simulink model "Quadrotor_Control"  (R2018b)
settings: Solver=VariableStepAuto  StartTime=0.0  StopTime=32  RelTol=1e-3
values from neighbouring files (symbols this model uses):
  d = 0.086    [lqrparameters.m]    (also in parameters.m = 0.25)
  g = 9.81    [lqrparameters.m]    (also in parameters.m)
  Ix = 0.00025    [lqrparameters.m]    (also in parameters.m)
  Iy = 0.000432    [lqrparameters.m]    (also in parameters.m)
  Iz = 0.0003738    [lqrparameters.m]    (also in parameters.m)
  kftx = 0.1    [lqrparameters.m]
  kfty = 0.1    [lqrparameters.m]
  kftz = 0.1    [lqrparameters.m]
  m = 0.18    [lqrparameters.m]    (also in parameters.m)
undefined symbols (not defined in the file or in its folder): DiscIntNeverNeededParam, K, kfax, kfay, kfaz
libraries: simulink x6
settings Model: Creator=Ayush  LastModifiedBy=Ayush

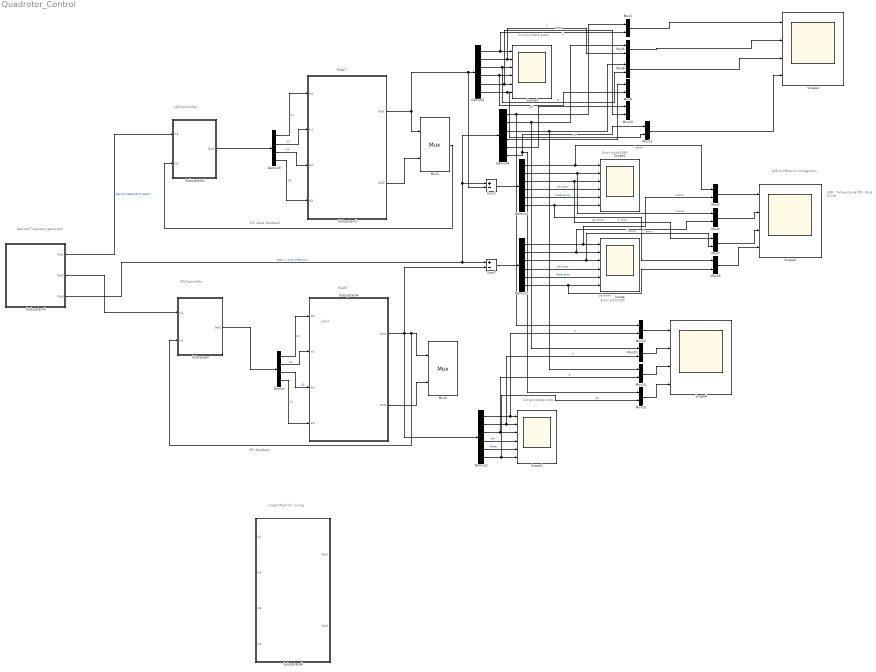
== system Quadrotor_Control ==
  note: Linear Plant for tuning
  note: LQR : Yellow Curve
      | PID : Blue Curve
  note: Desired Trajectory
      | generator
  note: PID
      | Controller
  note: PLANT
  note: Current State
      | plots
  note: PID feedback
  note: Error plots(LQR)
  note: LQR
      | Controller
  note: Full state feedback
  note: PLANT
  note: Current State
      | plots
  note: Error plots(PID)
  note: plant
  note: LQR vs PID
      | error comparison
  Demux : Demux
  Demux{1..2,4..6} (5 alike) : Demux  Outputs=6
  Demux3 : Demux
  Mux{1..16} (16 alike) : Mux  Inputs=2
      Mux1 settings: DisplayOption=signals
      Mux3 settings: DisplayOption=signals
  Scope{,1..3} (4 alike) : Scope  NumInputPorts=6
  Scope4 : Scope  NumInputPorts=4
  Scope5 : Scope  NumInputPorts=4
  Scope6 : Scope  NumInputPorts=4
  Subsystem : Subsystem
  Subsystem1 : Subsystem
  Subsystem2 : Subsystem
  Subsystem3 : Subsystem
  Subsystem4 : Subsystem
  Subsystem6 : Subsystem
  Sum1 : Sum  Inputs=+-
  Sum7 : Sum  Inputs=+-
  wires:
  Mux2/1 -> Scope5/1
  Mux7/1 -> Scope5/3
  Demux5/2 -> Mux6/2, Scope3/2  "Y"
  Demux3/2 -> Subsystem1/2(In1)  "U2"
  Demux5/4 -> Mux9/2, Scope3/4  "phi"
  Subsystem1/1(Out1) -> Mux1/1, Sum1/2, Demux5/1
  Demux4/6 -> Mux16/1, Scope2/6  "psi errror"
  Demux4/1 -> Mux2/1, Scope2/1  "X error"
  Sum1/1 -> Demux4/1
  Mux1/1 -> Subsystem2/2(In2)
  Subsystem2/1(Out1) -> Demux3/1
  Subsystem3/3(Out3) -> Demux6/1, Sum1/1, Sum7/1  "des(x,y,z,phi,theta,psi)"
  Demux3/1 -> Subsystem1/1(In5)  "U1"
  Demux5/3 -> Mux8/2, Scope3/3  "Z"
  Demux1/6 -> Mux16/2, Scope/6  "psi errror"
  Demux1/5 -> Scope/5  "theta error"
  Demux1/2 -> Mux4/2, Scope/2  "Y error"
  Demux3/3 -> Subsystem1/3(In2)  "U3"
  Demux4/5 -> Scope2/5  "theta error"
  Sum7/1 -> Demux1/1
  Mux4/1 -> Scope5/2
  Demux5/1 -> Mux5/2, Scope3/1  "X"
  Demux3/4 -> Subsystem1/4(In3)  "U4"
  Subsystem/1(Out1) -> Demux/1
  Subsystem3/1(Out1) -> Subsystem2/1(In1)  "des full state(12*1 vector)"
  Subsystem4/1(Out1) -> Sum7/2, Demux2/1, Subsystem/2(In2), Mux3/1
  Demux1/1 -> Mux2/2, Scope/1  "X error"
  Demux2/4 -> Scope1/4  "phi"
  Demux4/4 -> Scope2/4  "phi error"
  Demux2/1 -> Mux12/2, Scope1/1  "X"
  Demux4/3 -> Mux7/1, Scope2/3  "Z  error"
  Demux2/5 -> Scope1/5  "theta"
  Demux2/6 -> Mux15/2, Scope1/6  "psi"
  Demux5/6 -> Mux11/2, Scope3/6  "psi"
  Demux2/3 -> Mux14/2, Scope1/3  "Z"
  Demux1/3 -> Mux7/2, Scope/3  "Z  error"
  Demux4/2 -> Mux4/1, Scope2/2  "Y error"
  Demux2/2 -> Mux13/2, Scope1/2  "Y"
  Subsystem4/2(Out2) -> Mux3/2
  Demux1/4 -> Scope/4  "phi error"
  Demux5/5 -> Mux10/2, Scope3/5  "theta"
  Subsystem1/2(Out2) -> Mux1/2
  Demux6/1 -> Mux12/1, Mux5/1
  Demux6/2 -> Mux13/1, Mux6/1
  Demux6/3 -> Mux14/1, Mux8/1
  Demux6/4 -> Mux9/1
  Demux6/5 -> Mux10/1
  Demux6/6 -> Mux15/1, Mux11/1
  Mux6/1 -> Scope4/2
  Mux8/1 -> Scope4/3
  Mux5/1 -> Scope4/1
  Mux11/1 -> Scope4/4
  Mux12/1 -> Scope6/1
  Mux13/1 -> Scope6/2
  Mux14/1 -> Scope6/3
  Mux15/1 -> Scope6/4
  Mux16/1 -> Scope5/4
  Subsystem3/2(Out2) -> Subsystem/1(In1)
  Demux/1 -> Subsystem4/1(In5)  "U1"
  Demux/2 -> Subsystem4/2(In1)  "U2"
  Demux/3 -> Subsystem4/3(In2)  "U3"
  Demux/4 -> Subsystem4/4(In3)  "U4"

== system Quadrotor_Control/Subsystem ==
  note: attitude controller
  note: position controller
  In1 : Inport
  In2 : Inport  Port=2
  Demux : Demux  Outputs=6
  Demux1 : Demux
  Mux2 : Mux
  Subsystem2 : Subsystem
  Subsystem4 : Subsystem  Tag=Position Controller
  Out1 : Outport
  wires:
  Demux/1 -> Subsystem4/5(In5)  "X"
  Subsystem4/3(Out2) -> Subsystem2/1(In1)  "phi commanded"
  Demux1/4 -> Subsystem4/4(In4)  "psi des"
  Demux/5 -> Subsystem2/4(In4)  "theta"
  Subsystem4/4(Out4) -> Mux2/4  "U4"
  Demux1/1 -> Subsystem4/1(In1)  "x des"
  Subsystem4/1(Out3) -> Mux2/1  "U1"
  Subsystem2/1(Out1) -> Mux2/2  "U2"
  Subsystem4/2(Out1) -> Subsystem2/2(In2)  "theta commanded"
  Demux1/2 -> Subsystem4/2(In2)  "y des"
  Mux2/1 -> Out1/1
  Demux/2 -> Subsystem4/6(In6)  "Y"
  Subsystem2/2(Out2) -> Mux2/3  "U3"
  Demux/3 -> Subsystem4/7(In7)  "Z"
  Demux1/3 -> Subsystem4/3(In3)  "z des"
  Demux/4 -> Subsystem2/3(In3)  "phi"
  Demux/6 -> Subsystem4/8(In8)  "psi"
  In2/1 -> Demux/1  "Current State"
  In1/1 -> Demux1/1  "desired(x,y,z,psi)"

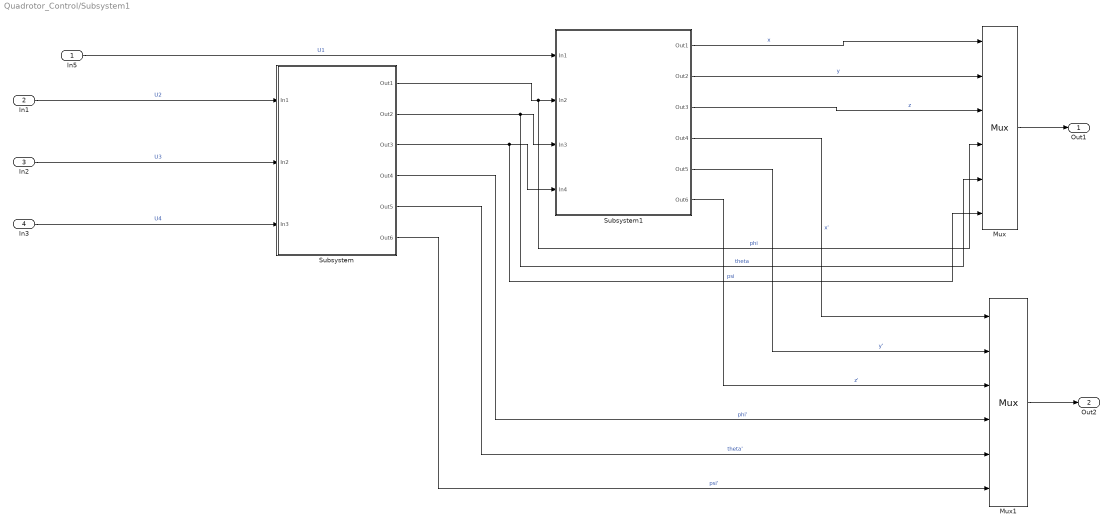
== system Quadrotor_Control/Subsystem1 ==
  In5 : Inport
  In1 : Inport  Port=2
  In2 : Inport  Port=3
  In3 : Inport  Port=4
  Mux : Mux  Inputs=6
      settings: DisplayOption=signals
  Mux1 : Mux  Inputs=6
      settings: DisplayOption=signals
  Subsystem : Subsystem
  Subsystem1 : Subsystem
  Out1 : Outport
  Out2 : Outport  Port=2
  wires:
  Subsystem1/2(Out2) -> Mux/2  "y"
  Subsystem/1(Out1) -> Subsystem1/2(In2), Mux/4  "phi"
  Subsystem1/1(Out1) -> Mux/1  "x"
  In1/1 -> Subsystem/1(In1)  "U2"
  Subsystem/3(Out3) -> Mux/6, Subsystem1/4(In4)  "psi"
  In3/1 -> Subsystem/3(In3)  "U4"
  Subsystem1/3(Out3) -> Mux/3  "z"
  Subsystem1/6(Out6) -> Mux1/3  "z'"
  In2/1 -> Subsystem/2(In2)  "U3"
  In5/1 -> Subsystem1/1(In1)  "U1"
  Subsystem1/4(Out4) -> Mux1/1  "x'"
  Subsystem1/5(Out5) -> Mux1/2  "y'"
  Subsystem/2(Out2) -> Mux/5, Subsystem1/3(In3)  "theta"
  Subsystem/4(Out4) -> Mux1/4  "phi'"
  Subsystem/5(Out5) -> Mux1/5  "theta'"
  Subsystem/6(Out6) -> Mux1/6  "psi'"
  Mux/1 -> Out1/1
  Mux1/1 -> Out2/1

== system Quadrotor_Control/Subsystem2 ==
  In1 : Inport
  In2 : Inport  Port=2
  Gain : Gain  Gain=K  Multiplication=Matrix(K*u)
  Sum : Sum  Inputs=+-
  Out1 : Outport
  wires:
  Sum/1 -> Gain/1
  Gain/1 -> Out1/1
  In1/1 -> Sum/1
  In2/1 -> Sum/2

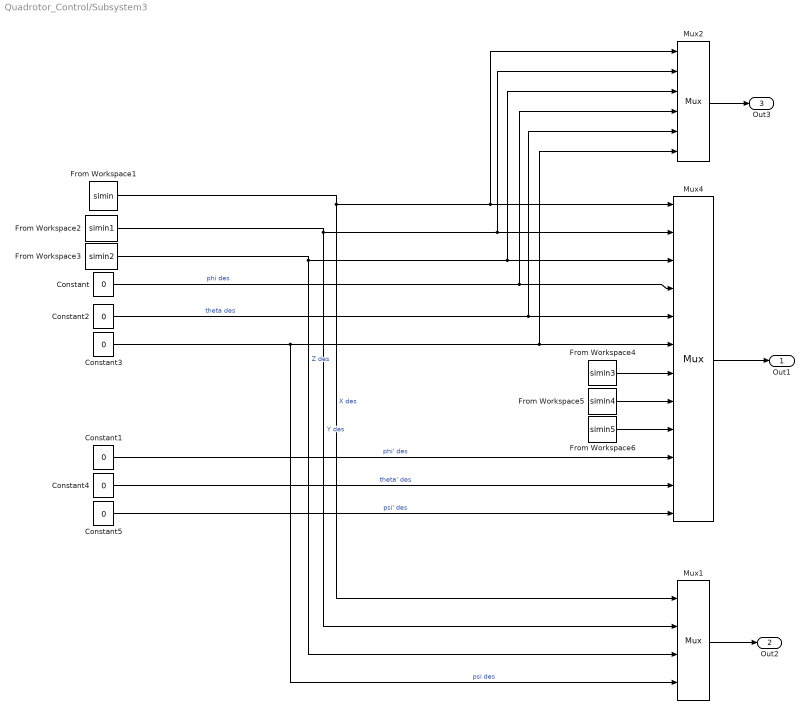
== system Quadrotor_Control/Subsystem3 ==
  Constant{,1..5} (6 alike) : Constant  Value=0
  From Workspace1 : FromWorkspace  VariableName=simin  SampleTime=0.001
  From Workspace2 : FromWorkspace  VariableName=simin1  SampleTime=0.001
  From Workspace3 : FromWorkspace  VariableName=simin2  SampleTime=0.001
  From Workspace4 : FromWorkspace  VariableName=simin3  SampleTime=0.001
  From Workspace5 : FromWorkspace  VariableName=simin4  SampleTime=0.001
  From Workspace6 : FromWorkspace  VariableName=simin5  SampleTime=0.001
  Mux1 : Mux
      settings: DisplayOption=signals
  Mux2 : Mux  Inputs=6
      settings: DisplayOption=signals
  Mux4 : Mux  Inputs=12
      settings: DisplayOption=signals
  Out1 : Outport
  Out2 : Outport  Port=2
  Out3 : Outport  Port=3
  wires:
  From Workspace1/1 -> Mux1/1, Mux2/1, Mux4/1  "X des"
  Constant1/1 -> Mux4/10  "phi' des"
  From Workspace2/1 -> Mux1/2, Mux2/2, Mux4/2  "Y des"
  Constant2/1 -> Mux2/5, Mux4/5  "theta des"
  Constant/1 -> Mux2/4, Mux4/4  "phi des"
  Constant5/1 -> Mux4/12  "psi' des"
  From Workspace3/1 -> Mux1/3, Mux2/3, Mux4/3  "Z des"
  Constant3/1 -> Mux1/4, Mux2/6, Mux4/6  "psi des"
  Constant4/1 -> Mux4/11  "theta' des"
  Mux1/1 -> Out2/1
  Mux4/1 -> Out1/1
  Mux2/1 -> Out3/1
  From Workspace4/1 -> Mux4/7
  From Workspace5/1 -> Mux4/8
  From Workspace6/1 -> Mux4/9

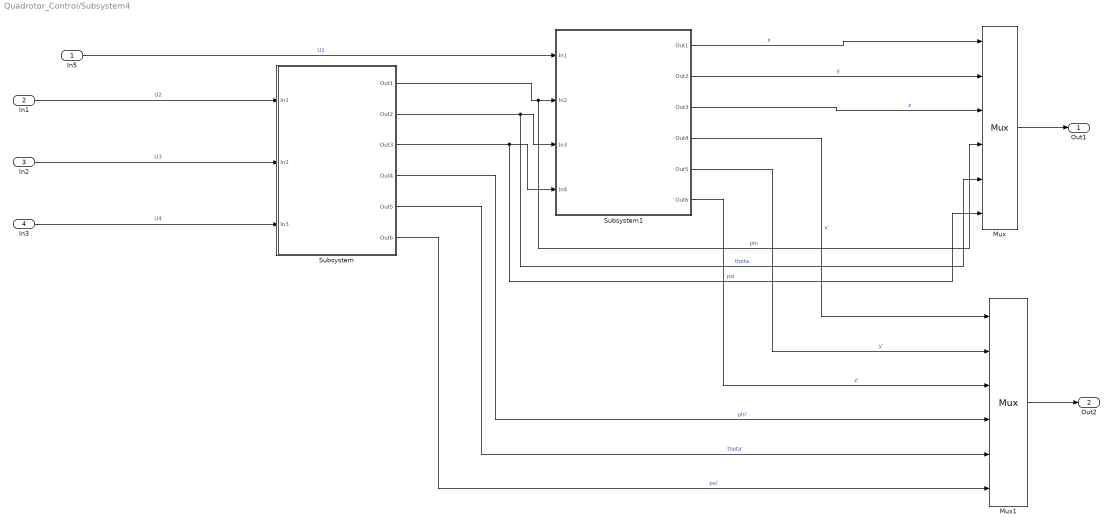
== system Quadrotor_Control/Subsystem4 ==
  In5 : Inport
  In1 : Inport  Port=2
  In2 : Inport  Port=3
  In3 : Inport  Port=4
  Mux : Mux  Inputs=6
      settings: DisplayOption=signals
  Mux1 : Mux  Inputs=6
      settings: DisplayOption=signals
  Subsystem : Subsystem
  Subsystem1 : Subsystem
  Out1 : Outport
  Out2 : Outport  Port=2
  wires:
  Subsystem1/2(Out2) -> Mux/2  "y"
  Subsystem/1(Out1) -> Subsystem1/2(In2), Mux/4  "phi"
  Subsystem1/1(Out1) -> Mux/1  "x"
  In1/1 -> Subsystem/1(In1)  "U2"
  Subsystem/3(Out3) -> Mux/6, Subsystem1/4(In4)  "psi"
  In3/1 -> Subsystem/3(In3)  "U4"
  Subsystem1/3(Out3) -> Mux/3  "z"
  Subsystem1/6(Out6) -> Mux1/3  "z'"
  In2/1 -> Subsystem/2(In2)  "U3"
  In5/1 -> Subsystem1/1(In1)  "U1"
  Subsystem1/4(Out4) -> Mux1/1  "x'"
  Subsystem1/5(Out5) -> Mux1/2  "y'"
  Subsystem/2(Out2) -> Mux/5, Subsystem1/3(In3)  "theta"
  Subsystem/4(Out4) -> Mux1/4  "phi'"
  Subsystem/5(Out5) -> Mux1/5  "theta'"
  Subsystem/6(Out6) -> Mux1/6  "psi'"
  Mux/1 -> Out1/1
  Mux1/1 -> Out2/1

== system Quadrotor_Control/Subsystem6 ==
  note: State Vector
      | Derivative
  note: State Vector
  In1 : Inport
  In2 : Inport  Port=2
  In3 : Inport  Port=3
  In4 : Inport  Port=4
  Mux1 : Mux  Inputs=6
      settings: DisplayOption=signals
  Mux3 : Mux  Inputs=6
      settings: DisplayOption=signals
  Subsystem1 : Subsystem
  Subsystem2 : Subsystem
  Out1 : Outport
  Out2 : Outport  Port=2
  wires:
  Subsystem1/1(Out1) -> Mux3/4, Subsystem2/2(In2)  "phi"
  Subsystem2/6(Out6) -> Mux1/3  "Z'"
  Subsystem2/5(Out5) -> Mux1/2  "Y'"
  Subsystem2/1(Out1) -> Mux3/1  "X"
  Subsystem1/2(Out2) -> Mux3/5, Subsystem2/3(In3)  "theta"
  Subsystem1/3(Out3) -> Mux3/6  "psi"
  Subsystem2/4(Out4) -> Mux1/1  "X'"
  Subsystem2/3(Out3) -> Mux3/3  "Z"
  In4/1 -> Subsystem1/3(In3)  "U4"
  In3/1 -> Subsystem1/2(In2)  "U3"
  Subsystem2/2(Out2) -> Mux3/2  "Y"
  In2/1 -> Subsystem1/1(In1)  "U2"
  In1/1 -> Subsystem2/1(In1)  "U1"
  Subsystem1/4(Out4) -> Mux1/4  "phi'"
  Subsystem1/5(Out5) -> Mux1/5  "theta'"
  Subsystem1/6(Out6) -> Mux1/6  "psi'"
  Mux1/1 -> Out2/1  "X' (State Derivative)"
  Mux3/1 -> Out1/1  "X(state Vector)"

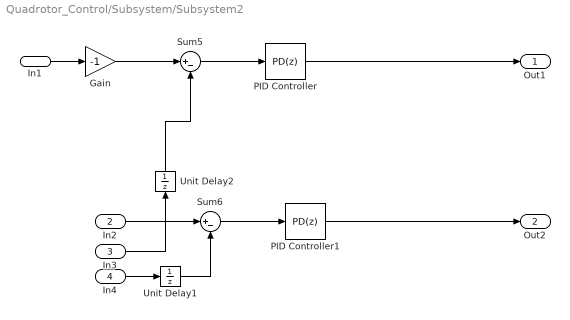
== system Quadrotor_Control/Subsystem/Subsystem2 ==
  In1 : Inport
  In2 : Inport  Port=2
  In3 : Inport  Port=3
  In4 : Inport  Port=4
  Gain : Gain  Gain=-1
  PID Controller : simulink/Continuous/PID Controller  Controller=PD  Form=Parallel  TimeDomain=Discrete-time  SampleTime=0.001  IntegratorMethod=Forward Euler  FilterMethod=Forward Euler  ControllerParametersSource=internal  P=0.492  I=0.1  D=0.08414  UseFilter=off  N=100  TunerSelectOption=Transfer Function Based (PID Tuner App)  InitialConditionSource=internal  InitialConditionForIntegrator=0  InitialConditionForFilter=0  DifferentiatorICPrevScaledInput=0  ExternalReset=none  TrackingMode=off  Kt=1  LimitOutput=off  UpperSaturationLimit=inf  LowerSaturationLimit=-inf  LinearizeAsGain=on  AntiWindupMode=none  Kb=1  POutMin=[]  POutMax=[]  IOutMin=[]  IOutMax=[]  DOutMin=[]  DOutMax=[]  NOutMin=[]  NOutMax=[]  SumOutMin=[]  SumOutMax=[]  SaturationOutMin=[]  SaturationOutMax=[]  PParamMin=[]  PParamMax=[]  IParamMin=[]  IParamMax=[]  DParamMin=[]  DParamMax=[]  NParamMin=[]  NParamMax=[]  KbParamMin=[]  KbParamMax=[]  KtParamMin=[]  KtParamMax=[]  KbOutMin=[]  KbOutMax=[]  KtOutMin=[]  KtOutMax=[]  IntegratorOutMin=[]  IntegratorOutMax=[]  FilterOutMin=[]  FilterOutMax=[]  SumI1OutMin=[]  SumI1OutMax=[]  SumI2OutMin=[]  SumI2OutMax=[]  SumI3OutMin=[]  SumI3OutMax=[]  SumI4OutMin=[]  SumI4OutMax=[]  SumDOutMin=[]  SumDOutMax=[]  DifferentiatorOutMin=[]  DifferentiatorOutMax=[]  FilterDiffOutCoefMin=[]  FilterDiffOutCoefMax=[]  ReciprocalOutMin=[]  ReciprocalOutMax=[]  SumDenOutMin=[]  SumDenOutMax=[]  SumNumOutMin=[]  SumNumOutMax=[]  DivideOutMin=[]  DivideOutMax=[]  IntegratorContinuousStateAttributes=''  IntegratorStateMustResolveToSignalObject=off  IntegratorRTWStateStorageClass=Auto  FilterContinuousStateAttributes=''  FilterStateMustResolveToSignalObject=off  FilterRTWStateStorageClass=Auto  ParallelPVariant=InternalParameters  IdealPVariant=Disabled  IVariant=Disabled  DVariant=InternalParameters  IntegratorVariant=Disabled  SatVariant=Disabled  AWVariant=Disabled  PCopyVariant=Disabled  TRVariant=Disabled  FdbkBlocksVariant=Forward  IdealPFdbkVariant=Disabled  SatFdbkVariant=Disabled  DerivativeFilterVariant=Differentiator  NVariant=Passthrough  NCopyVariant=Disabled_SignalSpec  FilterICVariant=InternalICsDifferentiator  IntegratorICVariant=Disabled  ExternalResetVariant=Disabled  TRSumVariant=Passthrough  SumFdbkVariant=Disabled  SumVariant=Sum_PD
  PID Controller1 : simulink/Continuous/PID Controller  Controller=PD  Form=Parallel  TimeDomain=Discrete-time  SampleTime=0.001  IntegratorMethod=Forward Euler  FilterMethod=Forward Euler  ControllerParametersSource=internal  P=0.7754  I=1  D=0.1389  UseFilter=off  N=100  TunerSelectOption=Transfer Function Based (PID Tuner App)  InitialConditionSource=internal  InitialConditionForIntegrator=0  InitialConditionForFilter=0  DifferentiatorICPrevScaledInput=0  ExternalReset=none  TrackingMode=off  Kt=1  LimitOutput=off  UpperSaturationLimit=inf  LowerSaturationLimit=-inf  LinearizeAsGain=on  AntiWindupMode=none  Kb=1  POutMin=[]  POutMax=[]  IOutMin=[]  IOutMax=[]  DOutMin=[]  DOutMax=[]  NOutMin=[]  NOutMax=[]  SumOutMin=[]  SumOutMax=[]  SaturationOutMin=[]  SaturationOutMax=[]  PParamMin=[]  PParamMax=[]  IParamMin=[]  IParamMax=[]  DParamMin=[]  DParamMax=[]  NParamMin=[]  NParamMax=[]  KbParamMin=[]  KbParamMax=[]  KtParamMin=[]  KtParamMax=[]  KbOutMin=[]  KbOutMax=[]  KtOutMin=[]  KtOutMax=[]  IntegratorOutMin=[]  IntegratorOutMax=[]  FilterOutMin=[]  FilterOutMax=[]  SumI1OutMin=[]  SumI1OutMax=[]  SumI2OutMin=[]  SumI2OutMax=[]  SumI3OutMin=[]  SumI3OutMax=[]  SumI4OutMin=[]  SumI4OutMax=[]  SumDOutMin=[]  SumDOutMax=[]  DifferentiatorOutMin=[]  DifferentiatorOutMax=[]  FilterDiffOutCoefMin=[]  FilterDiffOutCoefMax=[]  ReciprocalOutMin=[]  ReciprocalOutMax=[]  SumDenOutMin=[]  SumDenOutMax=[]  SumNumOutMin=[]  SumNumOutMax=[]  DivideOutMin=[]  DivideOutMax=[]  IntegratorContinuousStateAttributes=''  IntegratorStateMustResolveToSignalObject=off  IntegratorRTWStateStorageClass=Auto  FilterContinuousStateAttributes=''  FilterStateMustResolveToSignalObject=off  FilterRTWStateStorageClass=Auto  ParallelPVariant=InternalParameters  IdealPVariant=Disabled  IVariant=Disabled  DVariant=InternalParameters  IntegratorVariant=Disabled  SatVariant=Disabled  AWVariant=Disabled  PCopyVariant=Disabled  TRVariant=Disabled  FdbkBlocksVariant=Forward  IdealPFdbkVariant=Disabled  SatFdbkVariant=Disabled  DerivativeFilterVariant=Differentiator  NVariant=Passthrough  NCopyVariant=Disabled_SignalSpec  FilterICVariant=InternalICsDifferentiator  IntegratorICVariant=Disabled  ExternalResetVariant=Disabled  TRSumVariant=Passthrough  SumFdbkVariant=Disabled  SumVariant=Sum_PD
  Sum5 : Sum  Inputs=|+-
  Sum6 : Sum  Inputs=|+-
  Unit Delay1 : UnitDelay  SampleTime=0.001
  Unit Delay2 : UnitDelay  SampleTime=0.001
  Out1 : Outport
  Out2 : Outport  Port=2
  wires:
  Sum6/1 -> PID Controller1/1
  PID Controller1/1 -> Out2/1
  In2/1 -> Sum6/1
  In4/1 -> Unit Delay1/1
  Unit Delay1/1 -> Sum6/2
  PID Controller/1 -> Out1/1
  Sum5/1 -> PID Controller/1
  In1/1 -> Gain/1
  Gain/1 -> Sum5/1
  In3/1 -> Unit Delay2/1
  Unit Delay2/1 -> Sum5/2

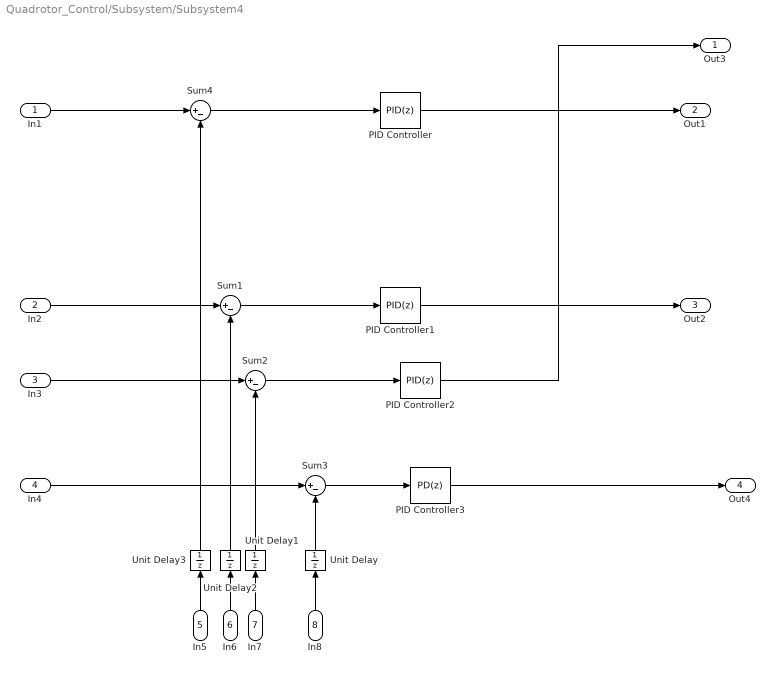
== system Quadrotor_Control/Subsystem/Subsystem4 ==
  In1 : Inport
  In2 : Inport  Port=2
  In3 : Inport  Port=3
  In4 : Inport  Port=4
  In5 : Inport  Port=5
  In6 : Inport  Port=6
  In7 : Inport  Port=7
  In8 : Inport  Port=8
  PID Controller : simulink/Continuous/PID Controller  Controller=PID  Form=Parallel  TimeDomain=Discrete-time  SampleTime=0.001  IntegratorMethod=Forward Euler  FilterMethod=Forward Euler  ControllerParametersSource=internal  P=0.4475  I=0.0442  D=1.133  UseFilter=off  N=100  TunerSelectOption=Transfer Function Based (PID Tuner App)  InitialConditionSource=internal  InitialConditionForIntegrator=0  InitialConditionForFilter=0  DifferentiatorICPrevScaledInput=0  ExternalReset=none  TrackingMode=off  Kt=1  LimitOutput=off  UpperSaturationLimit=inf  LowerSaturationLimit=-inf  LinearizeAsGain=on  AntiWindupMode=none  Kb=1  POutMin=[]  POutMax=[]  IOutMin=[]  IOutMax=[]  DOutMin=[]  DOutMax=[]  NOutMin=[]  NOutMax=[]  SumOutMin=[]  SumOutMax=[]  SaturationOutMin=[]  SaturationOutMax=[]  PParamMin=[]  PParamMax=[]  IParamMin=[]  IParamMax=[]  DParamMin=[]  DParamMax=[]  NParamMin=[]  NParamMax=[]  KbParamMin=[]  KbParamMax=[]  KtParamMin=[]  KtParamMax=[]  KbOutMin=[]  KbOutMax=[]  KtOutMin=[]  KtOutMax=[]  IntegratorOutMin=[]  IntegratorOutMax=[]  FilterOutMin=[]  FilterOutMax=[]  SumI1OutMin=[]  SumI1OutMax=[]  SumI2OutMin=[]  SumI2OutMax=[]  SumI3OutMin=[]  SumI3OutMax=[]  SumI4OutMin=[]  SumI4OutMax=[]  SumDOutMin=[]  SumDOutMax=[]  DifferentiatorOutMin=[]  DifferentiatorOutMax=[]  FilterDiffOutCoefMin=[]  FilterDiffOutCoefMax=[]  ReciprocalOutMin=[]  ReciprocalOutMax=[]  SumDenOutMin=[]  SumDenOutMax=[]  SumNumOutMin=[]  SumNumOutMax=[]  DivideOutMin=[]  DivideOutMax=[]  IntegratorContinuousStateAttributes=''  IntegratorStateMustResolveToSignalObject=off  IntegratorRTWStateStorageClass=Auto  FilterContinuousStateAttributes=''  FilterStateMustResolveToSignalObject=off  FilterRTWStateStorageClass=Auto  ParallelPVariant=InternalParameters  IdealPVariant=Disabled  IVariant=InternalParameters  DVariant=InternalParameters  IntegratorVariant=Discrete  SatVariant=Disabled  AWVariant=Passthrough  PCopyVariant=Disabled  TRVariant=Disabled  FdbkBlocksVariant=Forward  IdealPFdbkVariant=Disabled  SatFdbkVariant=Disabled  DerivativeFilterVariant=Differentiator  NVariant=Passthrough  NCopyVariant=Disabled_SignalSpec  FilterICVariant=InternalICsDifferentiator  IntegratorICVariant=InternalICs  ExternalResetVariant=Disabled  TRSumVariant=Passthrough  SumFdbkVariant=Disabled  SumVariant=Sum_PID
  PID Controller1 : simulink/Continuous/PID Controller  Controller=PID  Form=Parallel  TimeDomain=Discrete-time  SampleTime=0.001  IntegratorMethod=Forward Euler  FilterMethod=Forward Euler  ControllerParametersSource=internal  P=0.4473  I=0.04417  D=1.133  UseFilter=off  N=100  TunerSelectOption=Transfer Function Based (PID Tuner App)  InitialConditionSource=internal  InitialConditionForIntegrator=0  InitialConditionForFilter=0  DifferentiatorICPrevScaledInput=0  ExternalReset=none  TrackingMode=off  Kt=1  LimitOutput=off  UpperSaturationLimit=inf  LowerSaturationLimit=-inf  LinearizeAsGain=on  AntiWindupMode=none  Kb=1  POutMin=[]  POutMax=[]  IOutMin=[]  IOutMax=[]  DOutMin=[]  DOutMax=[]  NOutMin=[]  NOutMax=[]  SumOutMin=[]  SumOutMax=[]  SaturationOutMin=[]  SaturationOutMax=[]  PParamMin=[]  PParamMax=[]  IParamMin=[]  IParamMax=[]  DParamMin=[]  DParamMax=[]  NParamMin=[]  NParamMax=[]  KbParamMin=[]  KbParamMax=[]  KtParamMin=[]  KtParamMax=[]  KbOutMin=[]  KbOutMax=[]  KtOutMin=[]  KtOutMax=[]  IntegratorOutMin=[]  IntegratorOutMax=[]  FilterOutMin=[]  FilterOutMax=[]  SumI1OutMin=[]  SumI1OutMax=[]  SumI2OutMin=[]  SumI2OutMax=[]  SumI3OutMin=[]  SumI3OutMax=[]  SumI4OutMin=[]  SumI4OutMax=[]  SumDOutMin=[]  SumDOutMax=[]  DifferentiatorOutMin=[]  DifferentiatorOutMax=[]  FilterDiffOutCoefMin=[]  FilterDiffOutCoefMax=[]  ReciprocalOutMin=[]  ReciprocalOutMax=[]  SumDenOutMin=[]  SumDenOutMax=[]  SumNumOutMin=[]  SumNumOutMax=[]  DivideOutMin=[]  DivideOutMax=[]  IntegratorContinuousStateAttributes=''  IntegratorStateMustResolveToSignalObject=off  IntegratorRTWStateStorageClass=Auto  FilterContinuousStateAttributes=''  FilterStateMustResolveToSignalObject=off  FilterRTWStateStorageClass=Auto  ParallelPVariant=InternalParameters  IdealPVariant=Disabled  IVariant=InternalParameters  DVariant=InternalParameters  IntegratorVariant=Discrete  SatVariant=Disabled  AWVariant=Passthrough  PCopyVariant=Disabled  TRVariant=Disabled  FdbkBlocksVariant=Forward  IdealPFdbkVariant=Disabled  SatFdbkVariant=Disabled  DerivativeFilterVariant=Differentiator  NVariant=Passthrough  NCopyVariant=Disabled_SignalSpec  FilterICVariant=InternalICsDifferentiator  IntegratorICVariant=InternalICs  ExternalResetVariant=Disabled  TRSumVariant=Passthrough  SumFdbkVariant=Disabled  SumVariant=Sum_PID
  PID Controller2 : simulink/Continuous/PID Controller  Controller=PID  Form=Parallel  TimeDomain=Discrete-time  SampleTime=0.001  IntegratorMethod=Forward Euler  FilterMethod=Forward Euler  ControllerParametersSource=internal  P=0.8029  I=0.07931  D=2.032  UseFilter=off  N=100  TunerSelectOption=Transfer Function Based (PID Tuner App)  InitialConditionSource=internal  InitialConditionForIntegrator=0  InitialConditionForFilter=0  DifferentiatorICPrevScaledInput=0  ExternalReset=none  TrackingMode=off  Kt=1  LimitOutput=off  UpperSaturationLimit=inf  LowerSaturationLimit=-inf  LinearizeAsGain=on  AntiWindupMode=none  Kb=1  POutMin=[]  POutMax=[]  IOutMin=[]  IOutMax=[]  DOutMin=[]  DOutMax=[]  NOutMin=[]  NOutMax=[]  SumOutMin=[]  SumOutMax=[]  SaturationOutMin=[]  SaturationOutMax=[]  PParamMin=[]  PParamMax=[]  IParamMin=[]  IParamMax=[]  DParamMin=[]  DParamMax=[]  NParamMin=[]  NParamMax=[]  KbParamMin=[]  KbParamMax=[]  KtParamMin=[]  KtParamMax=[]  KbOutMin=[]  KbOutMax=[]  KtOutMin=[]  KtOutMax=[]  IntegratorOutMin=[]  IntegratorOutMax=[]  FilterOutMin=[]  FilterOutMax=[]  SumI1OutMin=[]  SumI1OutMax=[]  SumI2OutMin=[]  SumI2OutMax=[]  SumI3OutMin=[]  SumI3OutMax=[]  SumI4OutMin=[]  SumI4OutMax=[]  SumDOutMin=[]  SumDOutMax=[]  DifferentiatorOutMin=[]  DifferentiatorOutMax=[]  FilterDiffOutCoefMin=[]  FilterDiffOutCoefMax=[]  ReciprocalOutMin=[]  ReciprocalOutMax=[]  SumDenOutMin=[]  SumDenOutMax=[]  SumNumOutMin=[]  SumNumOutMax=[]  DivideOutMin=[]  DivideOutMax=[]  IntegratorContinuousStateAttributes=''  IntegratorStateMustResolveToSignalObject=off  IntegratorRTWStateStorageClass=Auto  FilterContinuousStateAttributes=''  FilterStateMustResolveToSignalObject=off  FilterRTWStateStorageClass=Auto  ParallelPVariant=InternalParameters  IdealPVariant=Disabled  IVariant=InternalParameters  DVariant=InternalParameters  IntegratorVariant=Discrete  SatVariant=Disabled  AWVariant=Passthrough  PCopyVariant=Disabled  TRVariant=Disabled  FdbkBlocksVariant=Forward  IdealPFdbkVariant=Disabled  SatFdbkVariant=Disabled  DerivativeFilterVariant=Differentiator  NVariant=Passthrough  NCopyVariant=Disabled_SignalSpec  FilterICVariant=InternalICsDifferentiator  IntegratorICVariant=InternalICs  ExternalResetVariant=Disabled  TRSumVariant=Passthrough  SumFdbkVariant=Disabled  SumVariant=Sum_PID
  PID Controller3 : simulink/Continuous/PID Controller  Controller=PD  Form=Parallel  TimeDomain=Discrete-time  SampleTime=0.001  IntegratorMethod=Forward Euler  FilterMethod=Forward Euler  ControllerParametersSource=internal  P=0.546  I=1  D=0.1077  UseFilter=off  N=100  TunerSelectOption=Transfer Function Based (PID Tuner App)  InitialConditionSource=internal  InitialConditionForIntegrator=0  InitialConditionForFilter=0  DifferentiatorICPrevScaledInput=0  ExternalReset=none  TrackingMode=off  Kt=1  LimitOutput=off  UpperSaturationLimit=inf  LowerSaturationLimit=-inf  LinearizeAsGain=on  AntiWindupMode=none  Kb=1  POutMin=[]  POutMax=[]  IOutMin=[]  IOutMax=[]  DOutMin=[]  DOutMax=[]  NOutMin=[]  NOutMax=[]  SumOutMin=[]  SumOutMax=[]  SaturationOutMin=[]  SaturationOutMax=[]  PParamMin=[]  PParamMax=[]  IParamMin=[]  IParamMax=[]  DParamMin=[]  DParamMax=[]  NParamMin=[]  NParamMax=[]  KbParamMin=[]  KbParamMax=[]  KtParamMin=[]  KtParamMax=[]  KbOutMin=[]  KbOutMax=[]  KtOutMin=[]  KtOutMax=[]  IntegratorOutMin=[]  IntegratorOutMax=[]  FilterOutMin=[]  FilterOutMax=[]  SumI1OutMin=[]  SumI1OutMax=[]  SumI2OutMin=[]  SumI2OutMax=[]  SumI3OutMin=[]  SumI3OutMax=[]  SumI4OutMin=[]  SumI4OutMax=[]  SumDOutMin=[]  SumDOutMax=[]  DifferentiatorOutMin=[]  DifferentiatorOutMax=[]  FilterDiffOutCoefMin=[]  FilterDiffOutCoefMax=[]  ReciprocalOutMin=[]  ReciprocalOutMax=[]  SumDenOutMin=[]  SumDenOutMax=[]  SumNumOutMin=[]  SumNumOutMax=[]  DivideOutMin=[]  DivideOutMax=[]  IntegratorContinuousStateAttributes=''  IntegratorStateMustResolveToSignalObject=off  IntegratorRTWStateStorageClass=Auto  FilterContinuousStateAttributes=''  FilterStateMustResolveToSignalObject=off  FilterRTWStateStorageClass=Auto  ParallelPVariant=InternalParameters  IdealPVariant=Disabled  IVariant=Disabled  DVariant=InternalParameters  IntegratorVariant=Disabled  SatVariant=Disabled  AWVariant=Disabled  PCopyVariant=Disabled  TRVariant=Disabled  FdbkBlocksVariant=Forward  IdealPFdbkVariant=Disabled  SatFdbkVariant=Disabled  DerivativeFilterVariant=Differentiator  NVariant=Passthrough  NCopyVariant=Disabled_SignalSpec  FilterICVariant=InternalICsDifferentiator  IntegratorICVariant=Disabled  ExternalResetVariant=Disabled  TRSumVariant=Passthrough  SumFdbkVariant=Disabled  SumVariant=Sum_PD
  Sum{1..4} (4 alike) : Sum  Inputs=|+-
  Unit Delay{,1..3} (4 alike) : UnitDelay  SampleTime=0.001
  Out3 : Outport
  Out1 : Outport  Port=2
  Out2 : Outport  Port=3
  Out4 : Outport  Port=4
  wires:
  PID Controller3/1 -> Out4/1
  In7/1 -> Unit Delay1/1
  In6/1 -> Unit Delay2/1
  In8/1 -> Unit Delay/1
  In5/1 -> Unit Delay3/1
  Unit Delay2/1 -> Sum1/2
  Sum1/1 -> PID Controller1/1
  Unit Delay1/1 -> Sum2/2
  Sum3/1 -> PID Controller3/1
  PID Controller1/1 -> Out2/1
  PID Controller2/1 -> Out3/1
  Sum2/1 -> PID Controller2/1
  Unit Delay/1 -> Sum3/2
  PID Controller/1 -> Out1/1
  Sum4/1 -> PID Controller/1
  Unit Delay3/1 -> Sum4/2
  In1/1 -> Sum4/1
  In2/1 -> Sum1/1
  In3/1 -> Sum2/1
  In4/1 -> Sum3/1

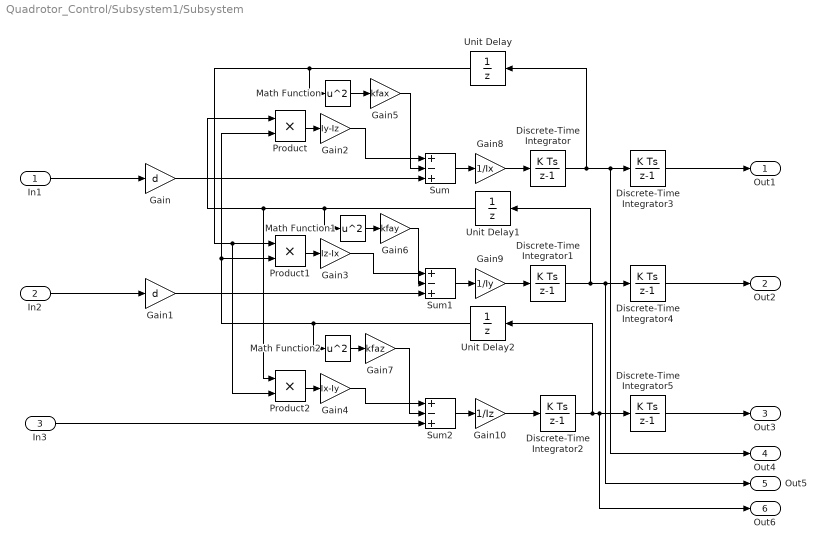
== system Quadrotor_Control/Subsystem1/Subsystem ==
  In1 : Inport
  In2 : Inport  Port=2
  In3 : Inport  Port=3
  Discrete-Time Integrator{,1..5} (6 alike) : DiscreteIntegrator  SampleTime=-1  ICPrevOutput=DiscIntNeverNeededParam  ICPrevScaledInput=DiscIntNeverNeededParam
  Gain : Gain  Gain=d
  Gain1 : Gain  Gain=d
  Gain10 : Gain  Gain=1/Iz
  Gain2 : Gain  Gain=Iy-Iz
  Gain3 : Gain  Gain=Iz-Ix
  Gain4 : Gain  Gain=Ix-Iy
  Gain5 : Gain  Gain=kfax
  Gain6 : Gain  Gain=kfay
  Gain7 : Gain  Gain=kfaz
  Gain8 : Gain  Gain=1/Ix
  Gain9 : Gain  Gain=1/Iy
  Math Function : Math  Operator=square  SaturateOnIntegerOverflow=on
  Math Function1 : Math  Operator=square  SaturateOnIntegerOverflow=on
  Math Function2 : Math  Operator=square  SaturateOnIntegerOverflow=on
  Product : Product
  Product1 : Product
  Product2 : Product
  Sum : Sum  Inputs=+-+
  Sum1 : Sum  Inputs=+-+
  Sum2 : Sum  Inputs=+-+
  Unit Delay : UnitDelay  SampleTime=0.001
  Unit Delay1 : UnitDelay  SampleTime=0.001
  Unit Delay2 : UnitDelay  SampleTime=0.001
  Out1 : Outport
  Out2 : Outport  Port=2
  Out3 : Outport  Port=3
  Out4 : Outport  Port=4
  Out5 : Outport  Port=5
  Out6 : Outport  Port=6
  wires:
  Unit Delay/1 -> Math Function/1, Product2/2, Product1/1
  Discrete-Time Integrator1/1 -> Out5/1, Discrete-Time Integrator4/1, Unit Delay1/1
  Unit Delay1/1 -> Math Function1/1, Product2/1, Product/1
  Discrete-Time Integrator2/1 -> Out6/1, Discrete-Time Integrator5/1, Unit Delay2/1
  Unit Delay2/1 -> Math Function2/1, Product1/2, Product/2
  Product1/1 -> Gain3/1
  Discrete-Time Integrator/1 -> Out4/1, Discrete-Time Integrator3/1, Unit Delay/1
  Gain10/1 -> Discrete-Time Integrator2/1
  Discrete-Time Integrator3/1 -> Out1/1
  Gain4/1 -> Sum2/1
  Gain/1 -> Sum/3
  Discrete-Time Integrator4/1 -> Out2/1
  Math Function/1 -> Gain5/1
  Gain5/1 -> Sum/2
  Product/1 -> Gain2/1
  Math Function1/1 -> Gain6/1
  Gain6/1 -> Sum1/2
  Gain7/1 -> Sum2/2
  Gain2/1 -> Sum/1
  Math Function2/1 -> Gain7/1
  Sum2/1 -> Gain10/1
  Gain9/1 -> Discrete-Time Integrator1/1
  Gain8/1 -> Discrete-Time Integrator/1
  Sum/1 -> Gain8/1
  Gain3/1 -> Sum1/1
  Product2/1 -> Gain4/1
  Gain1/1 -> Sum1/3
  Sum1/1 -> Gain9/1
  Discrete-Time Integrator5/1 -> Out3/1
  In1/1 -> Gain/1
  In2/1 -> Gain1/1
  In3/1 -> Sum2/3

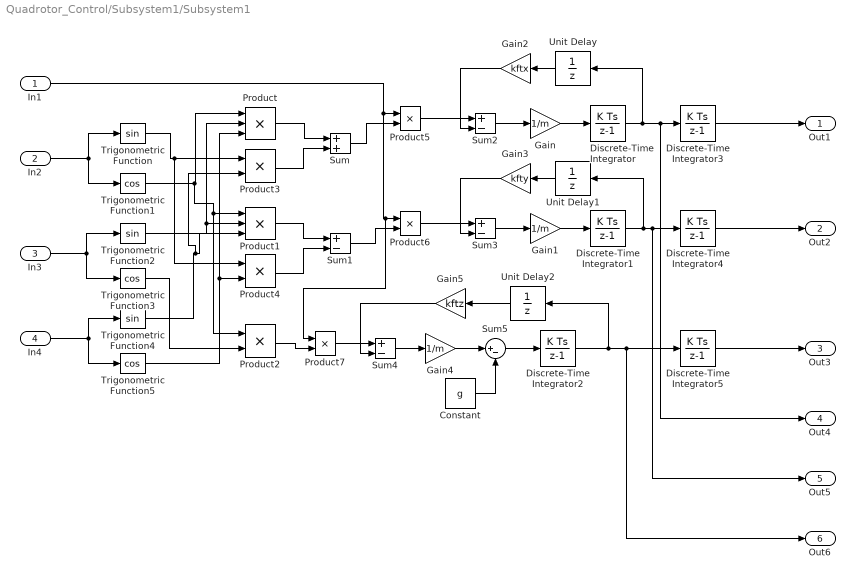
== system Quadrotor_Control/Subsystem1/Subsystem1 ==
  In1 : Inport
  In2 : Inport  Port=2
  In3 : Inport  Port=3
  In4 : Inport  Port=4
  Constant : Constant  Value=g
  Discrete-Time Integrator{,1..5} (6 alike) : DiscreteIntegrator  SampleTime=0.001  ICPrevOutput=DiscIntNeverNeededParam  ICPrevScaledInput=DiscIntNeverNeededParam
  Gain : Gain  Gain=1/m
  Gain1 : Gain  Gain=1/m
  Gain2 : Gain  Gain=kftx
  Gain3 : Gain  Gain=kfty
  Gain4 : Gain  Gain=1/m
  Gain5 : Gain  Gain=kftz
  Product : Product  Inputs=3
  Product1 : Product  Inputs=3
  Product{2..7} (6 alike) : Product
  Sum : Sum
  Sum{1..4} (4 alike) : Sum  Inputs=+-
  Sum5 : Sum  Inputs=|+-
  Trigonometric Function : Trigonometry
  Trigonometric Function1 : Trigonometry  Operator=cos
  Trigonometric Function2 : Trigonometry
  Trigonometric Function3 : Trigonometry  Operator=cos
  Trigonometric Function4 : Trigonometry
  Trigonometric Function5 : Trigonometry  Operator=cos
  Unit Delay : UnitDelay  SampleTime=0.001
  Unit Delay1 : UnitDelay  SampleTime=0.001
  Unit Delay2 : UnitDelay  SampleTime=0.001
  Out1 : Outport
  Out2 : Outport  Port=2
  Out3 : Outport  Port=3
  Out4 : Outport  Port=4
  Out5 : Outport  Port=5
  Out6 : Outport  Port=6
  wires:
  Sum2/1 -> Gain/1
  Trigonometric Function2/1 -> Product/2, Product1/2
  Unit Delay/1 -> Gain2/1
  Discrete-Time Integrator2/1 -> Out6/1, Discrete-Time Integrator5/1, Unit Delay2/1
  Gain5/1 -> Sum4/2
  Trigonometric Function4/1 -> Product3/2, Product1/3
  Trigonometric Function1/1 -> Product2/1, Product1/1, Product/1
  Product3/1 -> Sum/2
  Gain/1 -> Discrete-Time Integrator/1
  Product/1 -> Sum/1
  Sum5/1 -> Discrete-Time Integrator2/1
  Sum1/1 -> Product6/2
  Sum/1 -> Product5/2
  Product6/1 -> Sum3/1
  Discrete-Time Integrator1/1 -> Out5/1, Discrete-Time Integrator4/1, Unit Delay1/1
  In1/1 -> Product7/1, Product6/1, Product5/1
  Constant/1 -> Sum5/2
  Discrete-Time Integrator/1 -> Out4/1, Discrete-Time Integrator3/1, Unit Delay/1
  In3/1 -> Trigonometric Function2/1, Trigonometric Function3/1
  Sum4/1 -> Gain4/1
  Gain4/1 -> Sum5/1
  Unit Delay1/1 -> Gain3/1
  In4/1 -> Trigonometric Function5/1, Trigonometric Function4/1
  Trigonometric Function5/1 -> Product4/2, Product/3
  Trigonometric Function/1 -> Product4/1, Product3/1
  In2/1 -> Trigonometric Function1/1, Trigonometric Function/1
  Discrete-Time Integrator3/1 -> Out1/1
  Unit Delay2/1 -> Gain5/1
  Gain1/1 -> Discrete-Time Integrator1/1
  Sum3/1 -> Gain1/1
  Product5/1 -> Sum2/1
  Gain3/1 -> Sum3/2
  Gain2/1 -> Sum2/2
  Trigonometric Function3/1 -> Product2/2
  Product4/1 -> Sum1/2
  Product1/1 -> Sum1/1
  Discrete-Time Integrator4/1 -> Out2/1
  Discrete-Time Integrator5/1 -> Out3/1
  Product2/1 -> Product7/2
  Product7/1 -> Sum4/1

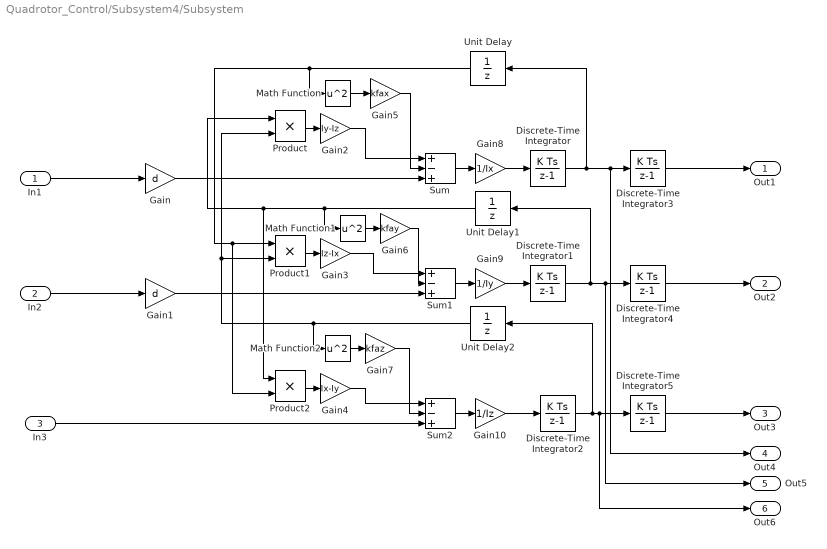
== system Quadrotor_Control/Subsystem4/Subsystem ==
  In1 : Inport
  In2 : Inport  Port=2
  In3 : Inport  Port=3
  Discrete-Time Integrator{,1..5} (6 alike) : DiscreteIntegrator  SampleTime=-1  ICPrevOutput=DiscIntNeverNeededParam  ICPrevScaledInput=DiscIntNeverNeededParam
  Gain : Gain  Gain=d
  Gain1 : Gain  Gain=d
  Gain10 : Gain  Gain=1/Iz
  Gain2 : Gain  Gain=Iy-Iz
  Gain3 : Gain  Gain=Iz-Ix
  Gain4 : Gain  Gain=Ix-Iy
  Gain5 : Gain  Gain=kfax
  Gain6 : Gain  Gain=kfay
  Gain7 : Gain  Gain=kfaz
  Gain8 : Gain  Gain=1/Ix
  Gain9 : Gain  Gain=1/Iy
  Math Function : Math  Operator=square  SaturateOnIntegerOverflow=on
  Math Function1 : Math  Operator=square  SaturateOnIntegerOverflow=on
  Math Function2 : Math  Operator=square  SaturateOnIntegerOverflow=on
  Product : Product
  Product1 : Product
  Product2 : Product
  Sum : Sum  Inputs=+-+
  Sum1 : Sum  Inputs=+-+
  Sum2 : Sum  Inputs=+-+
  Unit Delay : UnitDelay  SampleTime=0.001
  Unit Delay1 : UnitDelay  SampleTime=0.001
  Unit Delay2 : UnitDelay  SampleTime=0.001
  Out1 : Outport
  Out2 : Outport  Port=2
  Out3 : Outport  Port=3
  Out4 : Outport  Port=4
  Out5 : Outport  Port=5
  Out6 : Outport  Port=6
  wires:
  Unit Delay/1 -> Math Function/1, Product2/2, Product1/1
  Discrete-Time Integrator1/1 -> Out5/1, Discrete-Time Integrator4/1, Unit Delay1/1
  Unit Delay1/1 -> Math Function1/1, Product2/1, Product/1
  Discrete-Time Integrator2/1 -> Out6/1, Discrete-Time Integrator5/1, Unit Delay2/1
  Unit Delay2/1 -> Math Function2/1, Product1/2, Product/2
  Product1/1 -> Gain3/1
  Discrete-Time Integrator/1 -> Out4/1, Discrete-Time Integrator3/1, Unit Delay/1
  Gain10/1 -> Discrete-Time Integrator2/1
  Discrete-Time Integrator3/1 -> Out1/1
  Gain4/1 -> Sum2/1
  Gain/1 -> Sum/3
  Discrete-Time Integrator4/1 -> Out2/1
  Math Function/1 -> Gain5/1
  Gain5/1 -> Sum/2
  Product/1 -> Gain2/1
  Math Function1/1 -> Gain6/1
  Gain6/1 -> Sum1/2
  Gain7/1 -> Sum2/2
  Gain2/1 -> Sum/1
  Math Function2/1 -> Gain7/1
  Sum2/1 -> Gain10/1
  Gain9/1 -> Discrete-Time Integrator1/1
  Gain8/1 -> Discrete-Time Integrator/1
  Sum/1 -> Gain8/1
  Gain3/1 -> Sum1/1
  Product2/1 -> Gain4/1
  Gain1/1 -> Sum1/3
  Sum1/1 -> Gain9/1
  Discrete-Time Integrator5/1 -> Out3/1
  In1/1 -> Gain/1
  In2/1 -> Gain1/1
  In3/1 -> Sum2/3

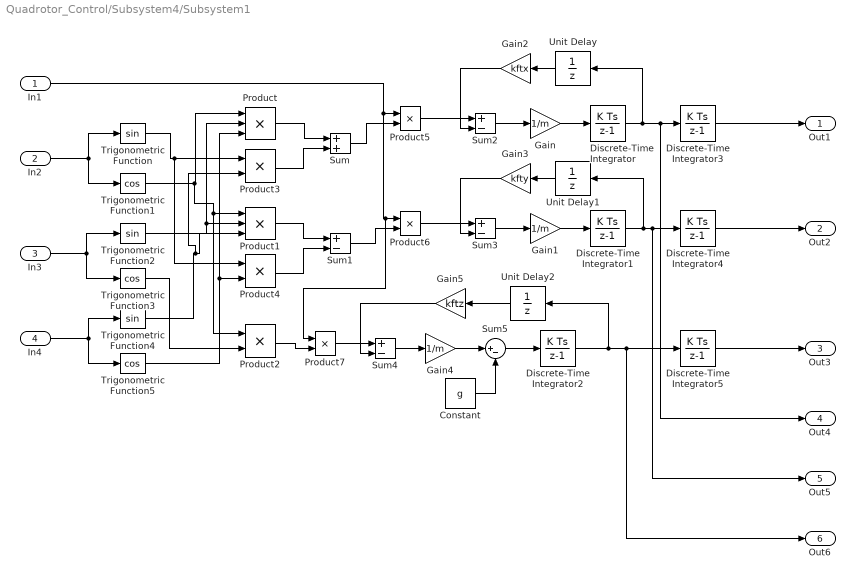
== system Quadrotor_Control/Subsystem4/Subsystem1 ==
  In1 : Inport
  In2 : Inport  Port=2
  In3 : Inport  Port=3
  In4 : Inport  Port=4
  Constant : Constant  Value=g
  Discrete-Time Integrator{,1..5} (6 alike) : DiscreteIntegrator  SampleTime=0.001  ICPrevOutput=DiscIntNeverNeededParam  ICPrevScaledInput=DiscIntNeverNeededParam
  Gain : Gain  Gain=1/m
  Gain1 : Gain  Gain=1/m
  Gain2 : Gain  Gain=kftx
  Gain3 : Gain  Gain=kfty
  Gain4 : Gain  Gain=1/m
  Gain5 : Gain  Gain=kftz
  Product : Product  Inputs=3
  Product1 : Product  Inputs=3
  Product{2..7} (6 alike) : Product
  Sum : Sum
  Sum{1..4} (4 alike) : Sum  Inputs=+-
  Sum5 : Sum  Inputs=|+-
  Trigonometric Function : Trigonometry
  Trigonometric Function1 : Trigonometry  Operator=cos
  Trigonometric Function2 : Trigonometry
  Trigonometric Function3 : Trigonometry  Operator=cos
  Trigonometric Function4 : Trigonometry
  Trigonometric Function5 : Trigonometry  Operator=cos
  Unit Delay : UnitDelay  SampleTime=0.001
  Unit Delay1 : UnitDelay  SampleTime=0.001
  Unit Delay2 : UnitDelay  SampleTime=0.001
  Out1 : Outport
  Out2 : Outport  Port=2
  Out3 : Outport  Port=3
  Out4 : Outport  Port=4
  Out5 : Outport  Port=5
  Out6 : Outport  Port=6
  wires:
  Sum2/1 -> Gain/1
  Trigonometric Function2/1 -> Product/2, Product1/2
  Unit Delay/1 -> Gain2/1
  Discrete-Time Integrator2/1 -> Out6/1, Discrete-Time Integrator5/1, Unit Delay2/1
  Gain5/1 -> Sum4/2
  Trigonometric Function4/1 -> Product3/2, Product1/3
  Trigonometric Function1/1 -> Product2/1, Product1/1, Product/1
  Product3/1 -> Sum/2
  Gain/1 -> Discrete-Time Integrator/1
  Product/1 -> Sum/1
  Sum5/1 -> Discrete-Time Integrator2/1
  Sum1/1 -> Product6/2
  Sum/1 -> Product5/2
  Product6/1 -> Sum3/1
  Discrete-Time Integrator1/1 -> Out5/1, Discrete-Time Integrator4/1, Unit Delay1/1
  In1/1 -> Product7/1, Product6/1, Product5/1
  Constant/1 -> Sum5/2
  Discrete-Time Integrator/1 -> Out4/1, Discrete-Time Integrator3/1, Unit Delay/1
  In3/1 -> Trigonometric Function2/1, Trigonometric Function3/1
  Sum4/1 -> Gain4/1
  Gain4/1 -> Sum5/1
  Unit Delay1/1 -> Gain3/1
  In4/1 -> Trigonometric Function5/1, Trigonometric Function4/1
  Trigonometric Function5/1 -> Product4/2, Product/3
  Trigonometric Function/1 -> Product4/1, Product3/1
  In2/1 -> Trigonometric Function1/1, Trigonometric Function/1
  Discrete-Time Integrator3/1 -> Out1/1
  Unit Delay2/1 -> Gain5/1
  Gain1/1 -> Discrete-Time Integrator1/1
  Sum3/1 -> Gain1/1
  Product5/1 -> Sum2/1
  Gain3/1 -> Sum3/2
  Gain2/1 -> Sum2/2
  Trigonometric Function3/1 -> Product2/2
  Product4/1 -> Sum1/2
  Product1/1 -> Sum1/1
  Discrete-Time Integrator4/1 -> Out2/1
  Discrete-Time Integrator5/1 -> Out3/1
  Product2/1 -> Product7/2
  Product7/1 -> Sum4/1

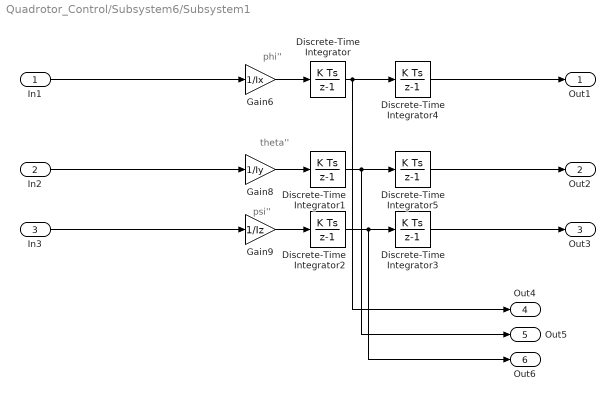
== system Quadrotor_Control/Subsystem6/Subsystem1 ==
  note: psi''
  note: theta''
  note: phi''
  In1 : Inport
  In2 : Inport  Port=2
  In3 : Inport  Port=3
  Discrete-Time Integrator{,1..5} (6 alike) : DiscreteIntegrator  SampleTime=0.001  ICPrevOutput=DiscIntNeverNeededParam  ICPrevScaledInput=DiscIntNeverNeededParam
  Gain6 : Gain  Gain=1/Ix
  Gain8 : Gain  Gain=1/Iy
  Gain9 : Gain  Gain=1/Iz
  Out1 : Outport
  Out2 : Outport  Port=2
  Out3 : Outport  Port=3
  Out4 : Outport  Port=4
  Out5 : Outport  Port=5
  Out6 : Outport  Port=6
  wires:
  Gain9/1 -> Discrete-Time Integrator2/1
  In2/1 -> Gain8/1
  Gain6/1 -> Discrete-Time Integrator/1
  Discrete-Time Integrator4/1 -> Out1/1
  Discrete-Time Integrator1/1 -> Out5/1, Discrete-Time Integrator5/1
  Discrete-Time Integrator5/1 -> Out2/1
  Gain8/1 -> Discrete-Time Integrator1/1
  Discrete-Time Integrator/1 -> Out4/1, Discrete-Time Integrator4/1
  Discrete-Time Integrator3/1 -> Out3/1
  In1/1 -> Gain6/1
  Discrete-Time Integrator2/1 -> Out6/1, Discrete-Time Integrator3/1
  In3/1 -> Gain9/1

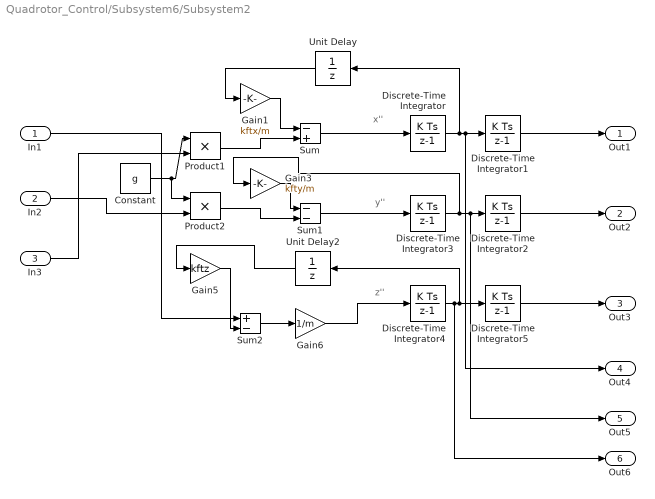
== system Quadrotor_Control/Subsystem6/Subsystem2 ==
  note: z''
  note: y''
  note: x''
  In1 : Inport
  In2 : Inport  Port=2
  In3 : Inport  Port=3
  Constant : Constant  Value=g  VectorParams1D=off
  Discrete-Time Integrator{,1..5} (6 alike) : DiscreteIntegrator  SampleTime=0.001  ICPrevOutput=DiscIntNeverNeededParam  ICPrevScaledInput=DiscIntNeverNeededParam
  Gain1 : Gain  Gain=kftx/m
  Gain3 : Gain  Gain=kfty/m
  Gain5 : Gain  Gain=kftz
  Gain6 : Gain  Gain=1/m
  Product1 : Product
  Product2 : Product
  Sum : Sum  Inputs=-+
  Sum1 : Sum  Inputs=--
  Sum2 : Sum  Inputs=+-
  Unit Delay : UnitDelay  SampleTime=0.001
  Unit Delay2 : UnitDelay  SampleTime=0.001
  Out1 : Outport
  Out2 : Outport  Port=2
  Out3 : Outport  Port=3
  Out4 : Outport  Port=4
  Out5 : Outport  Port=5
  Out6 : Outport  Port=6
  wires:
  Unit Delay/1 -> Gain1/1
  Discrete-Time Integrator/1 -> Out4/1, Discrete-Time Integrator1/1, Unit Delay/1
  Sum2/1 -> Gain6/1
  Unit Delay2/1 -> Gain5/1
  Discrete-Time Integrator5/1 -> Out3/1
  In1/1 -> Sum2/1
  Product1/1 -> Sum/2
  Gain5/1 -> Sum2/2
  Sum1/1 -> Discrete-Time Integrator3/1
  Discrete-Time Integrator4/1 -> Out6/1, Discrete-Time Integrator5/1, Unit Delay2/1
  Product2/1 -> Sum1/2
  Gain1/1 -> Sum/1
  Sum/1 -> Discrete-Time Integrator/1
  In3/1 -> Product1/2
  Discrete-Time Integrator3/1 -> Gain3/1, Out5/1, Discrete-Time Integrator2/1
  In2/1 -> Product2/2
  Gain3/1 -> Sum1/1
  Discrete-Time Integrator1/1 -> Out1/1
  Discrete-Time Integrator2/1 -> Out2/1
  Gain6/1 -> Discrete-Time Integrator4/1
  Constant/1 -> Product2/1, Product1/1
